simulink model "Classic_Sawmill"  (R2024b)
settings: Solver=FixedStepAuto  StartTime=0.0  StopTime=Tsim  FixedStep=dT  RelTol=1e-3
values from neighbouring files (symbols this model uses):
  b = t + 2*s    (= 3.6)    [ParametriSegheria.m]    (also in ParametriSegheriaDinamica.m; main_param_CLASSIC.m; main_param_SCADA.m)
  change_cost = 60    [ParametriSegheriaDinamica.m]    (also in main_param_CLASSIC.m = 50; main_param_SCADA.m = 50)
  dT = 0.025    [ParametriSegheriaDinamica.m]    (also in main_param_CLASSIC.m; main_param_SCADA.m)
  h_index = [70, 80, 90, 100]    [ParametriSegheria.m]    (also in ParametriSegheriaDinamica.m = [80, 90, 100]; main_param_CLASSIC.m = [80, 90, 100, 110]; main_param_SCADA.m = [80, 90, 100, 110])
  h_start_1 = 1    [main_param_CLASSIC.m]
  h_start_2 = 2    [main_param_CLASSIC.m]
  h_start_3 = 3    [main_param_CLASSIC.m]
  h_start_4 = 1    [main_param_CLASSIC.m]
  h_start_5 = 2    [main_param_CLASSIC.m]
  h_start_6 = 3    [main_param_CLASSIC.m]
  J1 = 8*1e6    (= 8000000)    [ParametriSegheriaDinamica.m]    (also in main_param_CLASSIC.m; main_param_SCADA.m)
  J2 = 0.9*1e6    (= 900000)    [ParametriSegheriaDinamica.m]    (also in main_param_CLASSIC.m; main_param_SCADA.m)
  kc = [0 35 40 50 55 90]    [ParametriSegheria.m]    (also in ParametriSegheriaDinamica.m = [0, 25, 30, 35, 50, 70]; main_param_CLASSIC.m = [0, 25, 30, 35, 50, 70]; main_param_SCADA.m = [0, 25, 30, 35, 50, 70])
  Kt = 2    [ParametriSegheria.m]    (also in ParametriSegheriaDinamica.m = 10000; main_param_CLASSIC.m = 10000; main_param_SCADA.m = 10000)
  Kt2 = 5    [ParametriSegheria.m]    (also in ParametriSegheriaDinamica.m = 4500; main_param_CLASSIC.m = 4500; main_param_SCADA.m = 4500)
  l_index = [20, 30, 40, 50]    [ParametriSegheria.m]    (also in ParametriSegheriaDinamica.m = [30, 40, 50]; main_param_CLASSIC.m = [30, 40, 50, 60]; main_param_SCADA.m = [30, 40, 50, 60])
  l_start_1 = 1    [main_param_CLASSIC.m]
  l_start_2 = 1    [main_param_CLASSIC.m]
  l_start_3 = 1    [main_param_CLASSIC.m]
  l_start_4 = 1    [main_param_CLASSIC.m]
  l_start_5 = 1    [main_param_CLASSIC.m]
  l_start_6 = 1    [main_param_CLASSIC.m]
  Lt = 4    [ParametriSegheria.m]    (also in ParametriSegheriaDinamica.m; main_param_CLASSIC.m; main_param_SCADA.m)
  Mag_D1 = [0 randi([220 500], 1, 40)]    [ParametriSegheria.m]    (also in ParametriSegheriaDinamica.m = [0 randi([200 500], 1, N_log)]; main_param_CLASSIC.m = [0 randi([200 500], 1, N_log)]; main_param_SCADA.m = [0 randi([200 500], 1, N_log)])
  Mag_D2 = [0 randi([220 500], 1, 40)]    [ParametriSegheria.m]    (also in ParametriSegheriaDinamica.m = [0 randi([200 500], 1, N_log)]; main_param_CLASSIC.m = [0 randi([200 500], 1, N_log)]; main_param_SCADA.m = [0 randi([200 500], 1, N_log)])
  Mag_D3 = [0 randi([220 500], 1, 40)]    [ParametriSegheria.m]    (also in ParametriSegheriaDinamica.m = [0 randi([200 500], 1, N_log)]; main_param_CLASSIC.m = [0 randi([200 500], 1, N_log)]; main_param_SCADA.m = [0 randi([200 500], 1, N_log)])
  Mag_legno1 = [0 randi([1 5], 1, 40)]    [ParametriSegheria.m]    (also in ParametriSegheriaDinamica.m = [0 randi([1 5], 1, N_log)]; main_param_CLASSIC.m = [0 randi([1 5], 1, N_log)]; main_param_SCADA.m = [0 randi([1 5], 1, N_log)])
  Mag_legno2 = [0 randi([1 5], 1, 40)]    [ParametriSegheria.m]    (also in ParametriSegheriaDinamica.m = [0 randi([1 5], 1, N_log)]; main_param_CLASSIC.m = [0 randi([1 5], 1, N_log)]; main_param_SCADA.m = [0 randi([1 5], 1, N_log)])
  Mag_legno3 = [0 randi([1 5], 1, 40)]    [ParametriSegheria.m]    (also in ParametriSegheriaDinamica.m = [0 randi([1 5], 1, N_log)]; main_param_CLASSIC.m = [0 randi([1 5], 1, N_log)]; main_param_SCADA.m = [0 randi([1 5], 1, N_log)])
  n_linee = 3    [ParametriSegheriaDinamica.m]    (also in main_param_CLASSIC.m; main_param_SCADA.m)
  omega_ref1 = 50    [ParametriSegheriaDinamica.m]    (also in main_param_CLASSIC.m; main_param_SCADA.m)
  omega_ref2 = 3000*(2*pi/60)    (= 314.159265359)    [ParametriSegheriaDinamica.m]    (also in main_param_CLASSIC.m; main_param_SCADA.m)
  Rc = 200    [ParametriSegheria.m]    (also in ParametriSegheriaDinamica.m; main_param_CLASSIC.m; main_param_SCADA.m)
  rho = [0, 450, 520, 590, 710, 780]*1e-9    [ParametriSegheriaDinamica.m]    (also in main_param_CLASSIC.m; main_param_SCADA.m)
  Rs = 800    [ParametriSegheria.m]    (also in ParametriSegheriaDinamica.m; main_param_CLASSIC.m; main_param_SCADA.m)
  sigma_D = 10    [ParametriSegheriaDinamica.m]    (also in main_param_CLASSIC.m = 5; main_param_SCADA.m = 5)
  sigma_larg = 10    [ParametriSegheriaDinamica.m]    (also in main_param_CLASSIC.m = 5; main_param_SCADA.m = 5)
  SR = Rs/Rm    (= 5.33333333333)    [ParametriSegheria.m]    (also in ParametriSegheriaDinamica.m; main_param_CLASSIC.m; main_param_SCADA.m)
  SR2 = Rc/Rm2    (= 4)    [ParametriSegheria.m]    (also in ParametriSegheriaDinamica.m; main_param_CLASSIC.m; main_param_SCADA.m)
  target_matrice = randi([20, 120], length(h_index), length(l_index))    [ParametriSegheria.m]    (also in ParametriSegheriaDinamica.m = randi([20, 100], length(h_index), length(l_index)); main_param_CLASSIC.m = randi([20, 100], length(h_index), length(l_index)); main_param_SCADA.m = randi([20, 100], length(h_index), length(l_index)))
  thr_lavoro = 600000    [ParametriSegheriaDinamica.m]    (also in main_param_CLASSIC.m; main_param_SCADA.m)
  V_mean1 = 0.75    [ParametriSegheriaDinamica.m]    (also in main_param_CLASSIC.m; main_param_SCADA.m)
  V_mean23 = 1    [ParametriSegheriaDinamica.m]    (also in main_param_CLASSIC.m; main_param_SCADA.m)
libraries: simulink x24, slpidlib x18
(part 4 of 5)

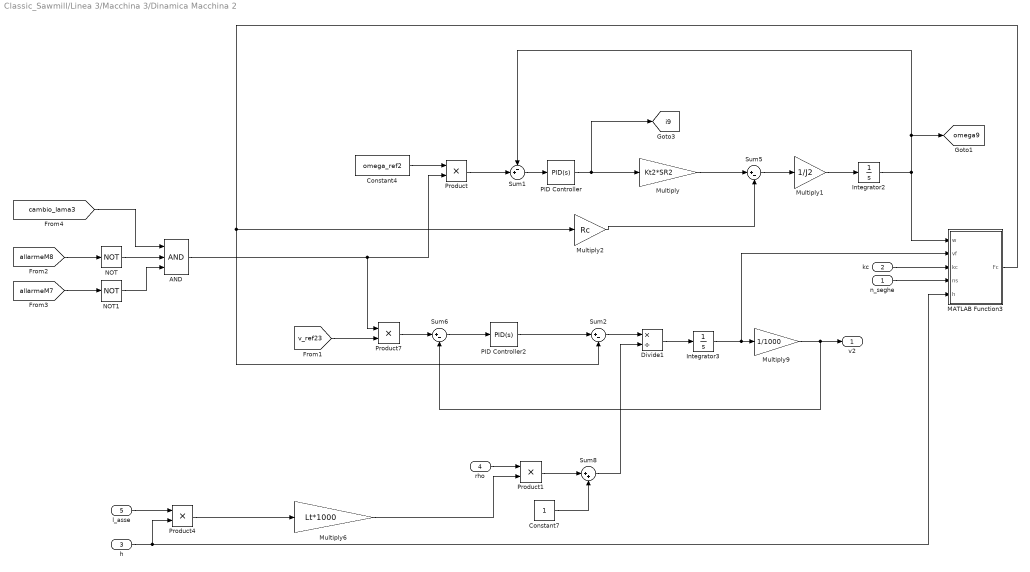
== system Classic_Sawmill/Linea 3/Macchina 3/Dinamica Macchina 2 ==
  n_seghe : Inport
  kc : Inport  Port=2
  h : Inport  Port=3
  rho : Inport  Port=4
  l_asse : Inport  Port=5
  AND : Logic  Inputs=3  IconShape=distinctive  AllPortsSameDT=off  OutDataTypeStr=boolean
  Constant4 : Constant  Value=omega_ref2
  Constant7 : Constant
  Divide1 : Product  Inputs=*/
  Integrator2 : Integrator  InitialCondition=omega_ref2
  Integrator3 : Integrator  InitialCondition=V_mean23*1000
  MATLAB Function3 : MATLAB Function  TreatAsAtomicUnit=on
  Multiply : Gain  Gain=Kt2*SR2
  Multiply1 : Gain  Gain=1/J2
  Multiply2 : Gain  Gain=Rc
  Multiply6 : Gain  Gain=Lt*1000
  Multiply9 : Gain  Gain=1/1000
  NOT : Logic  Operator=NOT  IconShape=distinctive  AllPortsSameDT=off  OutDataTypeStr=boolean
  NOT1 : Logic  Operator=NOT  IconShape=distinctive  AllPortsSameDT=off  OutDataTypeStr=boolean
  PID Controller : slpidlib/PID Controller  Controller=PID  Form=Parallel  TimeDomain=Continuous-time  UseExternalTs=off  SampleTime=-1  IntegratorMethod=Forward Euler  FilterMethod=Forward Euler  ControllerParametersSource=internal  P=345.484777327525  I=442.07289174245  UseKiTs=off  D=9.05690517196235  UseExternalDerivativeSource=off  N=26.4189049403583  UseFilter=on  TunerSelectOption=Transfer Function Based (PID Tuner App)  InitialConditionSource=internal  InitialConditionForIntegrator=0  InitialConditionForFilter=0  DifferentiatorICPrevScaledInput=0  ExternalReset=none  TrackingMode=off  Kt=1  LimitOutput=on  SatLimitsSource=internal  UpperSaturationLimit=300  LowerSaturationLimit=-300  LinearizeAsGain=on  AntiWindupMode=clamping  Kb=1  LimitIntegrator=off  UpperIntegratorSaturationLimit=200  LowerIntegratorSaturationLimit=-inf  POutMin=[]  POutMax=[]  IOutMin=[]  IOutMax=[]  DOutMin=[]  DOutMax=[]  NOutMin=[]  NOutMax=[]  SumOutMin=[]  SumOutMax=[]  SaturationOutMin=[]  SaturationOutMax=[]  PParamMin=[]  PParamMax=[]  IParamMin=[]  IParamMax=[]  DParamMin=[]  DParamMax=[]  NParamMin=[]  NParamMax=[]  KbParamMin=[]  KbParamMax=[]  KtParamMin=[]  KtParamMax=[]  KbOutMin=[]  KbOutMax=[]  KtOutMin=[]  KtOutMax=[]  IntegratorOutMin=[]  IntegratorOutMax=[]  FilterOutMin=[]  FilterOutMax=[]  SumI1OutMin=[]  SumI1OutMax=[]  SumI2OutMin=[]  SumI2OutMax=[]  SumI3OutMin=[]  SumI3OutMax=[]  SumI4OutMin=[]  SumI4OutMax=[]  SumDOutMin=[]  SumDOutMax=[]  DifferentiatorOutMin=[]  DifferentiatorOutMax=[]  FilterDiffOutCoefMin=[]  FilterDiffOutCoefMax=[]  ReciprocalOutMin=[]  ReciprocalOutMax=[]  SumDenOutMin=[]  SumDenOutMax=[]  SumNumOutMin=[]  SumNumOutMax=[]  DivideOutMin=[]  DivideOutMax=[]  UdiffTsProdOutMin=[]  UdiffTsProdOutMax=[]  NTsProdOutMin=[]  NTsProdOutMax=[]  UintegralTsProdOutMin=[]  UintegralTsProdOutMax=[]  UngainTsProdOutMin=[]  UngainTsProdOutMax=[]  ClampingZeroOutDataTypeStr=Inherit: Inherit via back propagation  ClampingZeroOutMin=[]  ClampingZeroOutMax=[]  FilterDenConstantOutDataTypeStr=Inherit: Inherit via back propagation  FilterDenConstantOutMin=[]  FilterDenConstantOutMax=[]  PCopyOutDataTypeStr=Inherit: Inherit via back propagation  PCopyOutMin=[]  PCopyOutMax=[]  NCopyOutDataTypeStr=Inherit: Inherit via back propagation  NCopyOutMin=[]  NCopyOutMax=[]  IntegratorContinuousStateAttributes=''  IntegratorStateMustResolveToSignalObject=off  IntegratorRTWStateStorageClass=Auto  FilterContinuousStateAttributes=''  FilterStateMustResolveToSignalObject=off  FilterRTWStateStorageClass=Auto  ParallelPVariant=InternalParameters  IdealPVariant=Disabled  IVariant=InternalParameters  DVariant=InternalParameters  IntegratorVariant=Continuous  SatVariant=Enabled  AWVariant=ContClampingParallel  PCopyVariant=Disabled  TRVariant=Disabled  FdbkBlocksVariant=Forward  IdealPFdbkVariant=Disabled  SatFdbkVariant=Disabled  DerivativeFilterVariant=ContFilter  NVariant=InternalParameters  NCopyVariant=Disabled  FilterICVariant=InternalICsFilter  IntegratorICVariant=InternalICs  ExternalResetVariant=Disabled  TRSumVariant=Passthrough  SumFdbkVariant=Disabled  SumVariant=Sum_PID  TsampFilterVariant=InternalTs  TsampNgainVariant=Passthrough  TsampIntegralVariant=Disabled_SignalSpec  ExternalSaturationOutDataTypeStr=Inherit: Same as second input  DerivativeSourceVariant=ErrorSignal  PreIntVariant=InternalPreInt
  PID Controller2 : slpidlib/PID Controller  Controller=PID  Form=Parallel  TimeDomain=Continuous-time  UseExternalTs=off  SampleTime=-1  IntegratorMethod=Forward Euler  FilterMethod=Forward Euler  ControllerParametersSource=internal  P=20866.9469532593  I=80635.0538109051  UseKiTs=off  D=181.138103439247  UseExternalDerivativeSource=off  N=79.7838174257724  UseFilter=on  TunerSelectOption=Transfer Function Based (PID Tuner App)  InitialConditionSource=internal  InitialConditionForIntegrator=0  InitialConditionForFilter=0  DifferentiatorICPrevScaledInput=0  ExternalReset=none  TrackingMode=off  Kt=1  LimitOutput=on  SatLimitsSource=internal  UpperSaturationLimit=5000  LowerSaturationLimit=-5000  LinearizeAsGain=off  AntiWindupMode=clamping  Kb=1  LimitIntegrator=off  UpperIntegratorSaturationLimit=200  LowerIntegratorSaturationLimit=-inf  POutMin=[]  POutMax=[]  IOutMin=[]  IOutMax=[]  DOutMin=[]  DOutMax=[]  NOutMin=[]  NOutMax=[]  SumOutMin=[]  SumOutMax=[]  SaturationOutMin=[]  SaturationOutMax=[]  PParamMin=[]  PParamMax=[]  IParamMin=[]  IParamMax=[]  DParamMin=[]  DParamMax=[]  NParamMin=[]  NParamMax=[]  KbParamMin=[]  KbParamMax=[]  KtParamMin=[]  KtParamMax=[]  KbOutMin=[]  KbOutMax=[]  KtOutMin=[]  KtOutMax=[]  IntegratorOutMin=[]  IntegratorOutMax=[]  FilterOutMin=[]  FilterOutMax=[]  SumI1OutMin=[]  SumI1OutMax=[]  SumI2OutMin=[]  SumI2OutMax=[]  SumI3OutMin=[]  SumI3OutMax=[]  SumI4OutMin=[]  SumI4OutMax=[]  SumDOutMin=[]  SumDOutMax=[]  DifferentiatorOutMin=[]  DifferentiatorOutMax=[]  FilterDiffOutCoefMin=[]  FilterDiffOutCoefMax=[]  ReciprocalOutMin=[]  ReciprocalOutMax=[]  SumDenOutMin=[]  SumDenOutMax=[]  SumNumOutMin=[]  SumNumOutMax=[]  DivideOutMin=[]  DivideOutMax=[]  UdiffTsProdOutMin=[]  UdiffTsProdOutMax=[]  NTsProdOutMin=[]  NTsProdOutMax=[]  UintegralTsProdOutMin=[]  UintegralTsProdOutMax=[]  UngainTsProdOutMin=[]  UngainTsProdOutMax=[]  ClampingZeroOutDataTypeStr=Inherit: Inherit via back propagation  ClampingZeroOutMin=[]  ClampingZeroOutMax=[]  FilterDenConstantOutDataTypeStr=Inherit: Inherit via back propagation  FilterDenConstantOutMin=[]  FilterDenConstantOutMax=[]  PCopyOutDataTypeStr=Inherit: Inherit via back propagation  PCopyOutMin=[]  PCopyOutMax=[]  NCopyOutDataTypeStr=Inherit: Inherit via back propagation  NCopyOutMin=[]  NCopyOutMax=[]  IntegratorContinuousStateAttributes=''  IntegratorStateMustResolveToSignalObject=off  IntegratorRTWStateStorageClass=Auto  FilterContinuousStateAttributes=''  FilterStateMustResolveToSignalObject=off  FilterRTWStateStorageClass=Auto  ParallelPVariant=InternalParameters  IdealPVariant=Disabled  IVariant=InternalParameters  DVariant=InternalParameters  IntegratorVariant=Continuous  SatVariant=Enabled  AWVariant=ContClampingParallel  PCopyVariant=Disabled  TRVariant=Disabled  FdbkBlocksVariant=Forward  IdealPFdbkVariant=Disabled  SatFdbkVariant=Disabled  DerivativeFilterVariant=ContFilter  NVariant=InternalParameters  NCopyVariant=Disabled  FilterICVariant=InternalICsFilter  IntegratorICVariant=InternalICs  ExternalResetVariant=Disabled  TRSumVariant=Passthrough  SumFdbkVariant=Disabled  SumVariant=Sum_PID  TsampFilterVariant=InternalTs  TsampNgainVariant=Passthrough  TsampIntegralVariant=Disabled_SignalSpec  ExternalSaturationOutDataTypeStr=Inherit: Same as second input  DerivativeSourceVariant=ErrorSignal  PreIntVariant=InternalPreInt
  Product{,1,4,7} (4 alike) : Product
  Sum1 : Sum  Inputs=-+|
  Sum2 : Sum  Inputs=|+-
  Sum5 : Sum  Inputs=|+-
  Sum6 : Sum  Inputs=|+-
  Sum8 : Sum  Inputs=|++
  v2 : Outport
  tag scope: i9=global, omega9=global
  wires:
  Product4/1 -> Multiply6/1
  h/1 -> MATLAB Function3/5(h), Product4/2
  l_asse/1 -> Product4/1
  Constant4/1 -> Product/1
  [v_ref23] -> Product7/2
  Product/1 -> Sum1/2
  Sum1/1 -> PID Controller/1
  rho/1 -> Product1/1
  AND/1 -> Product/2, Product7/1
  Sum5/1 -> Multiply1/1
  Multiply1/1 -> Integrator2/1
  PID Controller/1 -> [i9], Multiply/1
  MATLAB Function3/1(Fc) -> Sum2/2, Multiply2/1
  Sum6/1 -> PID Controller2/1
  Divide1/1 -> Integrator3/1
  Integrator3/1 -> MATLAB Function3/2(vf), Multiply9/1
  PID Controller2/1 -> Sum2/1
  Integrator2/1 -> MATLAB Function3/1(w), [omega9], Sum1/1
  Sum2/1 -> Divide1/1
  Product7/1 -> Sum6/1
  kc/1 -> MATLAB Function3/3(kc)
  Multiply6/1 -> Product1/2
  n_seghe/1 -> MATLAB Function3/4(ns)
  Product1/1 -> Sum8/1
  Sum8/1 -> Divide1/2
  Constant7/1 -> Sum8/2
  Multiply9/1 -> v2/1, Sum6/2
  Multiply/1 -> Sum5/1
  Multiply2/1 -> Sum5/2
  NOT1/1 -> AND/3
  [allarmeM8] -> NOT/1
  [allarmeM7] -> NOT1/1
  NOT/1 -> AND/2
  [cambio_lama3] -> AND/1

== matlab function Classic_Sawmill/Linea 1/MATLAB Function1 ==
  data: u input; y output
function y = fcn(u)

    persistent n_prec

    if isempty(n_prec)
        n_prec = 0;
    end

    y = u - n_prec;

    n_prec = u;

== matlab function Classic_Sawmill/Controllo Magazzino/MATLAB Function4 ==
  data: u input; idx output; h_index parameter
function idx = find_index(u, h_index)
%#codegen

v = h_index;

idx = -1; % valore default se non trovato

for i = 1:length(v)
    if u == v(i)
        idx = i;
        return;
    end
end

== matlab function Classic_Sawmill/Controllo Magazzino/MATLAB Function5 ==
  data: u input; idx output; l_index parameter
function idx = find_index(u, l_index)
%#codegen

v = l_index;

idx = -1; % valore default se non trovato

for i = 1:length(v)
    if u == v(i)
        idx = i;
        return;
    end
end

== matlab function Classic_Sawmill/Linea 2/MATLAB Function ==
  data: u input; y output
function y = fcn(u)

    persistent n_prec

    if isempty(n_prec)
        n_prec = 0;
    end

    y = u - n_prec;


    n_prec = u;

== matlab function Classic_Sawmill/Linea 2/MATLAB Function1 ==
  data: u input; y output
function y = fcn(u)

    persistent n_prec

    if isempty(n_prec)
        n_prec = 0;
    end

    y = u - n_prec;

    n_prec = u;

== matlab function Classic_Sawmill/Linea 2/MATLAB Function2 ==
  settings: updateMethod=DISCRETE
  data: lama_usurata input; y output; tronco_finito input
function y = fcn(lama_usurata, tronco_finito)
    
    persistent cambia_lama
    if isempty(cambia_lama)
        cambia_lama = 0;
    end

    if lama_usurata == 1
        cambia_lama = 1;
    end

    if tronco_finito == 1 && cambia_lama == 1
        y = cambia_lama;
        cambia_lama = 0;
    else
        y = 0;
    end

== matlab function Classic_Sawmill/Linea 2/MATLAB Function3 ==
  settings: updateMethod=DISCRETE
  data: u input; y output; t input; tempo_cambio parameter
function y = f(u, t, tempo_cambio)
persistent t_start active

if isempty(active)
    active = false;
    t_start = 0;
end

if u == 1 && ~active
    t_start = t;
    active = true;
end

if active
    if (t - t_start) <= tempo_cambio
        y = 0;
    else
        y = 1;
        active = false;
    end
else
    y = 1;
end

== matlab function Classic_Sawmill/Linea 2/Macchina 1/Dinamica Macchina 1/MATLAB Function3 ==
  data: w input; Fc output; vf input; kc input; Dt input; Rs parameter; b parameter
function Fc = Fcfun(w, vf, kc, Dt, Rs, b)

if w < 0.01
    Fc = 0;
else
    Fc = kc*b*vf*Dt/(w*Rs);
end

== matlab function Classic_Sawmill/Linea 2/Macchina 1/Logica Macchina 1/MATLAB Function ==
  data: u input; y output; Mag_legno2 parameter
function y = fcn(u, Mag_legno2)
    persistent counter
    if isempty(counter)
        counter = 1;
    end

    if u == 1
        counter = counter + 1;
    end

    y = counter;
    
    if y > length(Mag_legno2)-1
        y = 0;
    end

end

== matlab function Classic_Sawmill/Linea 3/MATLAB Function ==
  data: u input; y output
function y = fcn(u)

    persistent n_prec

    if isempty(n_prec)
        n_prec = 0;
    end

    y = u - n_prec;


    n_prec = u;

== matlab function Classic_Sawmill/Linea 3/MATLAB Function1 ==
  data: u input; y output
function y = fcn(u)

    persistent n_prec

    if isempty(n_prec)
        n_prec = 0;
    end

    y = u - n_prec;

    n_prec = u;

== matlab function Classic_Sawmill/Linea 3/MATLAB Function2 ==
  settings: updateMethod=DISCRETE
  data: lama_usurata input; y output; tronco_finito input
function y = fcn(lama_usurata, tronco_finito)
    
    persistent cambia_lama
    if isempty(cambia_lama)
        cambia_lama = 0;
    end

    if lama_usurata == 1
        cambia_lama = 1;
    end

    if tronco_finito == 1 && cambia_lama == 1
        y = cambia_lama;
        cambia_lama = 0;
    else
        y = 0;
    end

== matlab function Classic_Sawmill/Linea 3/MATLAB Function3 ==
  settings: updateMethod=DISCRETE
  data: u input; y output; t input; tempo_cambio parameter
function y = f(u, t,tempo_cambio)
persistent t_start active

if isempty(active)
    active = false;
    t_start = 0;
end

if u == 1 && ~active
    t_start = t;
    active = true;
end

if active
    if (t - t_start) <= tempo_cambio
        y = 0;
    else
        y = 1;
        active = false;
    end
else
    y = 1;
end

== matlab function Classic_Sawmill/Linea 3/Macchina 1/Dinamica Macchina 1/MATLAB Function3 ==
  data: w input; Fc output; vf input; kc input; Dt input; Rs parameter; b parameter
function Fc = Fcfun(w, vf, kc, Dt, Rs, b)

if w < 0.01
    Fc = 0;
else
    Fc = kc*b*vf*Dt/(w*Rs);
end

== matlab function Classic_Sawmill/Linea 3/Macchina 1/Logica Macchina 1/MATLAB Function ==
  data: u input; y output; Mag_legno3 parameter
function y = fcn(u, Mag_legno3)
    persistent counter
    if isempty(counter)
        counter = 1;
    end

    if u == 1
        counter = counter + 1;
    end

    y = counter;
    
    if y > length(Mag_legno3)-1
        y = 0;
    end

end

== matlab function Classic_Sawmill/Controllo Magazzino/MATLAB Function6 ==
  data: u input; idx output; h_index parameter
function idx = find_index(u, h_index)
%#codegen

v = h_index;

idx = -1; % valore default se non trovato

for i = 1:length(v)
    if u == v(i)
        idx = i;
        return;
    end
end

== matlab function Classic_Sawmill/Controllo Magazzino/MATLAB Function7 ==
  data: u input; idx output; h_index parameter
function idx = find_index(u, h_index)
%#codegen

v = h_index;

idx = -1; % valore default se non trovato

for i = 1:length(v)
    if u == v(i)
        idx = i;
        return;
    end
end

== matlab function Classic_Sawmill/Controllo Magazzino/MATLAB Function8 ==
  data: u input; idx output; h_index parameter
function idx = find_index(u, h_index)
%#codegen

v = h_index;

idx = -1; % valore default se non trovato

for i = 1:length(v)
    if u == v(i)
        idx = i;
        return;
    end
end

== matlab function Classic_Sawmill/Controllo Magazzino/MATLAB Function9 ==
  data: u input; idx output; h_index parameter
function idx = find_index(u, h_index)
%#codegen

v = h_index;

idx = -1; % valore default se non trovato

for i = 1:length(v)
    if u == v(i)
        idx = i;
        return;
    end
end

== matlab function Classic_Sawmill/Controllo Magazzino/MATLAB Function10 ==
  data: u input; idx output; l_index parameter
function idx = find_index(u, l_index)
%#codegen

v = l_index;

idx = -1; % valore default se non trovato

for i = 1:length(v)
    if u == v(i)
        idx = i;
        return;
    end
end

== matlab function Classic_Sawmill/Controllo Magazzino/MATLAB Function11 ==
  data: u input; idx output; l_index parameter
function idx = find_index(u, l_index)
%#codegen

v = l_index;

idx = -1; % valore default se non trovato

for i = 1:length(v)
    if u == v(i)
        idx = i;
        return;
    end
end

== matlab function Classic_Sawmill/Controllo Magazzino/MATLAB Function12 ==
  data: u input; idx output; l_index parameter
function idx = find_index(u, l_index)
%#codegen

v = l_index;

idx = -1; % valore default se non trovato

for i = 1:length(v)
    if u == v(i)
        idx = i;
        return;
    end
end

== matlab function Classic_Sawmill/Controllo Magazzino/MATLAB Function13 ==
  data: u input; idx output; l_index parameter
function idx = find_index(u, l_index)
%#codegen

v = l_index;

idx = -1; % valore default se non trovato

for i = 1:length(v)
    if u == v(i)
        idx = i;
        return;
    end
end

== matlab function Classic_Sawmill/Controllo Magazzino/INTELLIGENTE ==
  data: h_next output; Magazzino output; stop output; l_next output; h_idx input; target_matrice parameter; n_assi input; l_idx input; change_cost parameter; flag output
function [h_next, Magazzino, stop, l_next, flag] = fcn(h_idx, target_matrice, n_assi, l_idx, change_cost)

[n_rows, n_cols] = size(target_matrice);

h_next = zeros(1,length(h_idx));
l_next = zeros(1,length(l_idx));

persistent MagazzinoReale



if isempty(MagazzinoReale)
    MagazzinoReale = zeros(n_rows, n_cols);
end

for i = 1:length(n_assi)
    % Output iniziali
    h_next(i) = h_idx(i);
    l_next(i) = l_idx(i);
    

    MagazzinoReale(h_idx(i), l_idx(i)) = MagazzinoReale(h_idx(i), l_idx(i)) + n_assi(i);
end
    

% AVVISO QUANDO STO PER FINIRE QUELLA SEZIONE
thr = 10;
diff = zeros(1, length(n_assi));
flag = zeros(1, length(n_assi));

for i = 1:length(n_assi)
    diff(i) = target_matrice(h_idx(i), l_idx(i)) - MagazzinoReale(h_idx(i), l_idx(i));
    if diff(i) <= thr
        flag(i) = 1;
    else 
        flag(i) = 0;
    end
end



for i = 1:length(n_assi)
    if MagazzinoReale(h_idx(i), l_idx(i)) >= target_matrice(h_idx(i), l_idx(i)) + 1


        deficit = target_matrice - MagazzinoReale;

        best_cost = inf;
        best_h = h_idx(i);
        best_l = l_idx(i);

        
        for h = 1:n_rows
            for l = 1:n_cols

                if deficit(h,l) > 0

                    % Penalità cambio lama
                    if mod(i, 2) == 0
                        cambio = (h ~= h_idx(i));
                    else
                        cambio = (l ~= l_idx(i));
                    end

                    % Funzione costo
                    cost = -deficit(h,l) + change_cost*cambio;

                    if cost < best_cost
                        best_cost = cost;
                        best_h = h;
                        best_l = l;
                    end
                end

            end
        end

        if best_cost < inf
            h_next(i) = best_h;
            l_next(i) = best_l;
        end

    end
end

if MagazzinoReale >= target_matrice
    stop = 1;
else
    stop = 0;
end

Magazzino = MagazzinoReale;

== matlab function Classic_Sawmill/Linea 3/Macchina 1/Logica Macchina 1/MATLAB Function2 ==
  settings: updateMethod=DISCRETE
  data: spessore input; u input; spessore2 input; diametro input; y output; larg_asse output; thickness output; finito output; prior output; likelihood output; posterior output; larg_stim output; sigma_post output; sigma_larg parameter; sigma_D parameter
function [y, larg_asse, thickness, finito, prior, likelihood, posterior, larg_stim, sigma_post]= fcn(spessore, u, spessore2, diametro, sigma_larg, sigma_D)
    
    persistent in_rnd
        
    if isempty(in_rnd)
        rng(42, "twister");
        in_rnd = true;
    end

    persistent counter

    persistent noise_D

    if isempty(noise_D)
        noise_D = sigma_D*randn();
    end
  
    thin_cut = 4;

    max_assi = floor((diametro-thin_cut*spessore2) / spessore);
    finito = 0;

    maxD = 1000;
    larg_vec = 0:maxD;

    prior = zeros(size(larg_vec));
    likelihood = zeros(size(larg_vec));
    posterior = zeros(size(larg_vec));

    if isempty(counter)
        counter = 0;
    end
    

    % Conto assi tagliate
    if u == 1
        counter = counter + 1;
    end

    % Quando finisco tronco segnalo e azzero counter
    if counter > max_assi + thin_cut
        finito = 1;
        counter = 0;
    end

    if finito ~= 0
        noise_D = sigma_D*randn();
    end
    
    if diametro > 0
        misure_D = diametro + noise_D;
    else
        misure_D = diametro;
    end

    % SISTEMARE INCERTEZZA: propagata da D in L
    if counter == 0
        larg_asse = 0;
        larg_asseD = 0;
        thickness = 0;
        sigma_largD = 0;
    elseif counter <= thin_cut/2
        distanza_bordo = counter * spessore2;
        larg_asse = sqrt((diametro)^2-(spessore2 + diametro - 2*distanza_bordo)^2);
        thickness = spessore2;
        % prior
        larg_asseD = sqrt(abs((misure_D)^2-(spessore2 + misure_D - 2*distanza_bordo)^2));
        sigma_largD = abs((2*distanza_bordo - spessore2)/sqrt((2*distanza_bordo - spessore2)*(-2*distanza_bordo + 2*diametro + spessore2)))*sigma_D;
    elseif counter > max_assi + thin_cut/2
        distanza_bordo = max_assi*spessore + (counter-max_assi)*spessore2;
        larg_asse = sqrt((diametro)^2-(spessore2 + diametro - 2*distanza_bordo)^2);
        thickness = spessore2;
        % prior
        larg_asseD = sqrt(abs((misure_D)^2-(spessore2 + misure_D - 2*distanza_bordo)^2));
        sigma_largD = abs((2*distanza_bordo - spessore2)/sqrt((2*distanza_bordo - spessore2)*(-2*distanza_bordo + 2*diametro + spessore2)))*sigma_D;
    else
        % Calcolo larghezza delle assi
        distanza_bordo = thin_cut/2 * spessore2 + (counter-thin_cut/2) * spessore;
        larg_asse = sqrt((diametro)^2-(spessore + diametro - 2*distanza_bordo)^2);
        thickness = spessore;
        % prior
        larg_asseD = sqrt(abs((misure_D)^2-(spessore + misure_D - 2*distanza_bordo)^2));
        sigma_largD = abs((2*distanza_bordo - spessore)/sqrt((2*distanza_bordo - spessore)*(-2*distanza_bordo + 2*diametro + spessore)))*sigma_D;
    end




    if larg_asse > 0
        misure_larg = larg_asse + sigma_larg * randn();
    else
        misure_larg = larg_asse;
    end

    if larg_asse > 0
        prior(:) = 1/sqrt(2*pi*sigma_largD^2)*exp(-0.5 * ((larg_vec - larg_asseD) / sigma_largD).^2);
        prior(:) = prior(:) / sum(prior(:));
    else
        prior(:) = 0;
    end

    if misure_larg > 0
        likelihood(:) = 1/sqrt(2*pi*sigma_larg^2)*exp(-0.5 * ((larg_vec - misure_larg) / sigma_larg).^2);
        likelihood(:) = likelihood(:) / sum(likelihood(:));
    else
        likelihood(:) = 0;
    end

    if misure_larg > 0 && larg_asse > 0
        posterior(:) = prior(:) .* likelihood(:);
        posterior(:) = posterior(:) / sum(posterior(:));
    else
        posterior(:) = 0;
    end



    [~, idx] = max(posterior(:)); 

    larg_stim = larg_vec(idx);
    % (sigma_likelihood^2*sigma_prior^2)/(sigma_likelihood^2 + sigma_prior^2)
    sigma_post = sqrt( (sigma_largD^2*sigma_larg^2) / (sigma_largD^2 + sigma_larg^2) );
    
    y = counter;

== matlab function Classic_Sawmill/Controllo Magazzino/CAMBIO LAME CONSUMATE ==
  data: n_assi input; y output; cambio_1 output; cambio_2 output; cambio_3 output; kc input; Lt parameter; b parameter; h input; lavoro_l output; thr_lavoro parameter
function [y, cambio_1, cambio_2, cambio_3, lavoro_l] = fcn(n_assi, kc, Lt, b,h, thr_lavoro)

    warning = zeros(1, length(n_assi));

    persistent usura_lama
    persistent lavoro_lama

    if isempty(usura_lama)
        usura_lama = zeros(1, length(n_assi));
    end

    if isempty(lavoro_lama)
        lavoro_lama = zeros(1, length(n_assi));
    end

    cambio_1 = 0;
    cambio_2 = 0;
    cambio_3 = 0;

    for i = 1:length(n_assi)
        
        % Ogni volta che arriva un certo numero di assi vuol dire che le
        % lame hanno appena fatto un taglio
        if n_assi(i) ~= 0
            usura_lama(i) = usura_lama(i) + 1;
            lavoro_lama(i) = lavoro_lama(i) + kc(i)*b*Lt*h(i);
        end
        
        if lavoro_lama(i) > thr_lavoro
            warning(i) = 1;
            lavoro_lama(i) = 0;
        end

        % i = 1 -> M2 Linea 1
        % i = 2 -> M3 Linea 1
        % i = 3 -> M2 Linea 2
        % i = 4 -> M3 Linea 2
        % i = 5 -> M2 Linea 3
        % i = 6 -> M2 Linea 3
        if (i == 1 || i == 2) && warning(i) == 1
            cambio_1 = 1;
        elseif (i == 3 || i == 4) && warning(i) == 1
            cambio_2 = 1;
        elseif (i == 5 || i == 6) && warning(i) == 1
            cambio_3 = 1;
        end

    end

    lavoro_l = lavoro_lama;

    y = warning;

== matlab function Classic_Sawmill/Linea 1/Macchina 2/Dinamica Macchina 2/MATLAB Function3 ==
  data: w input; Fc output; vf input; kc input; ns input; h input; Rs parameter; b parameter
function Fc = Fcfun(w, vf, kc, ns, h, Rs, b)

if w < 0.01
    Fc = 0;
else
    Fc = ns*kc*b*vf*h/(w*Rs);
end

== matlab function Classic_Sawmill/Linea 1/MATLAB Function3 ==
  settings: updateMethod=DISCRETE
  data: u input; y output; t input; tempo_cambio parameter
function y = f(u, t, tempo_cambio)
persistent t_start active

if isempty(active)
    active = false;
    t_start = 0;
end

if u == 1 && ~active
    t_start = t;
    active = true;
end

if active
    if (t - t_start) <= tempo_cambio
        y = 0;
    else
        y = 1;
        active = false;
    end
else
    y = 1;
end

== matlab function Classic_Sawmill/Linea 1/Macchina 1/Logica Macchina 1/MATLAB Function1 ==
  settings: updateMethod=DISCRETE
  data: spessore input; u input; spessore2 input; diametro input; y output; larg_asse output; thickness output; finito output; prior output; likelihood output; posterior output; larg_stim output; sigma_post output; sigma_larg parameter; sigma_D parameter; t input
function [y, larg_asse, thickness, finito, prior, likelihood, posterior, larg_stim, sigma_post]= fcn(spessore, u, spessore2, diametro, sigma_larg, sigma_D, t)
    
    persistent in_rnd
        
    if isempty(in_rnd)
        rng(42, "twister");
        in_rnd = true;
    end

    persistent counter

    persistent noise_D

    if isempty(noise_D)
        noise_D = sigma_D*randn();
    end
  
    thin_cut = 4;

    max_assi = floor((diametro-thin_cut*spessore2) / spessore);
    finito = 0;

    maxD = 1000;
    larg_vec = 0:maxD;

    prior = zeros(size(larg_vec));
    likelihood = zeros(size(larg_vec));
    posterior = zeros(size(larg_vec));

    if isempty(counter)
        counter = 0;
    end
    

    % Conto assi tagliate
    if u == 1
        counter = counter + 1;
    end

    % Quando finisco tronco segnalo e azzero counter
    if counter > max_assi + thin_cut
        finito = 1;
        counter = 0;
    end

    if finito ~= 0
        noise_D = sigma_D*randn();
    end
    
    if diametro > 0
        misure_D = diametro + noise_D;
    else
        misure_D = diametro;
    end

    % SISTEMARE INCERTEZZA: propagata da D in L
    if counter == 0
        larg_asse = 0;
        larg_asseD = 0;
        thickness = 0;
        sigma_largD = 0;
        distanza_bordo = 0;
    elseif counter <= thin_cut/2
        distanza_bordo = counter * spessore2;
        larg_asse = sqrt((diametro)^2-(spessore2 + diametro - 2*distanza_bordo)^2);
        thickness = spessore2;
        % prior
        larg_asseD = sqrt(abs((misure_D)^2-(spessore2 + misure_D - 2*distanza_bordo)^2));
        sigma_largD = abs((2*distanza_bordo - spessore2)/sqrt((2*distanza_bordo - spessore2)*(-2*distanza_bordo + 2*diametro + spessore2)))*sigma_D;
    elseif counter > max_assi + thin_cut/2
        distanza_bordo = max_assi*spessore + (counter-max_assi)*spessore2;
        larg_asse = sqrt((diametro)^2-(spessore2 + diametro - 2*distanza_bordo)^2);
        thickness = spessore2;
        % prior
        larg_asseD = sqrt(abs((misure_D)^2-(spessore2 + misure_D - 2*distanza_bordo)^2));
        sigma_largD = abs((2*distanza_bordo - spessore2)/sqrt((2*distanza_bordo - spessore2)*(-2*distanza_bordo + 2*diametro + spessore2)))*sigma_D;
    else
        % Calcolo larghezza delle assi
        distanza_bordo = thin_cut/2 * spessore2 + (counter-thin_cut/2) * spessore;
        larg_asse = sqrt((diametro)^2-(spessore + diametro - 2*distanza_bordo)^2);
        thickness = spessore;
        % prior
        larg_asseD = sqrt(abs((misure_D)^2-(spessore + misure_D - 2*distanza_bordo)^2));
        sigma_largD = abs((2*distanza_bordo - spessore)/sqrt((2*distanza_bordo - spessore)*(-2*distanza_bordo + 2*diametro + spessore)))*sigma_D;
    end


    sens_break = 0;

    if larg_asse > 0
        if t > 35 && t < 50 && sens_break
            misure_larg = larg_asse + sigma_larg * randn() + 100*rand;
        else
            misure_larg = larg_asse + sigma_larg * randn();
        end
    else
        misure_larg = larg_asse;
    end

    if larg_asse > 0
        prior(:) = 1/sqrt(2*pi*sigma_largD^2)*exp(-0.5 * ((larg_vec - larg_asseD) / sigma_largD).^2);
        prior(:) = prior(:) / sum(prior(:));
    else
        prior(:) = 0;
    end

    if misure_larg > 0
        likelihood(:) = 1/sqrt(2*pi*sigma_larg^2)*exp(-0.5 * ((larg_vec - misure_larg) / sigma_larg).^2);
        likelihood(:) = likelihood(:) / sum(likelihood(:));
    else
        likelihood(:) = 0;
    end

    if misure_larg > 0 && larg_asse > 0
        posterior(:) = prior(:) .* likelihood(:);
        posterior(:) = posterior(:) / sum(posterior(:));
    else
        posterior(:) = 0;
    end



    [~, idx] = max(posterior(:)); 

    larg_stim = larg_vec(idx);
    % (sigma_likelihood^2*sigma_prior^2)/(sigma_likelihood^2 + sigma_prior^2)
    sigma_post = sqrt( (sigma_largD^2*sigma_larg^2) / (sigma_largD^2 + sigma_larg^2) );
    
    y = counter;

== matlab function Classic_Sawmill/Linea 2/Macchina 2/Dinamica Macchina 2/MATLAB Function3 ==
  data: w input; Fc output; vf input; kc input; ns input; h input; Rs parameter; b parameter
function Fc = Fcfun(w, vf, kc, ns, h, Rs, b)

if w < 0.01
    Fc = 0;
else
    Fc = ns*kc*b*vf*h/(w*Rs);
end

== matlab function Classic_Sawmill/Linea 1/Macchina 2/MATLAB Function2 ==
  settings: updateMethod=DISCRETE
  data: u input; w_asse input; y output; l_asse input; taglio output; Lt parameter
function [y, taglio] = fcn(u, w_asse, l_asse,Lt)
    persistent counter 

    n_assi = floor(l_asse / w_asse);
    
    taglio = 0;

    if isempty(counter)
        counter = 0;
    end

    % Conto assi tagliate
    if u >= Lt
        counter = counter + n_assi;
    end

    % Segnale di taglio
    if  (u > 0 && u < Lt && l_asse > 0) 
        taglio = 1;
    end
    y = counter;
end

== matlab function Classic_Sawmill/Linea 3/Macchina 2/Dinamica Macchina 2/MATLAB Function3 ==
  data: w input; Fc output; vf input; kc input; ns input; h input; Rs parameter; b parameter
function Fc = Fcfun(w, vf, kc, ns, h, Rs, b)

if w < 0.01
    Fc = 0;
else
    Fc = ns*kc*b*vf*h/(w*Rs);
end

== matlab function Classic_Sawmill/Linea 1/Macchina 3/Dinamica Macchina 2/MATLAB Function3 ==
  data: w input; Fc output; vf input; kc input; ns input; h input; Rs parameter; b parameter
function Fc = Fcfun(w, vf, kc, ns, h, Rs, b)

if w < 0.01
    Fc = 0;
else
    Fc = ns*kc*b*vf*h/(w*Rs);
end

== matlab function Classic_Sawmill/Linea 1/Macchina 3/MATLAB Function2 ==
  settings: updateMethod=DISCRETE
  data: u input; w_asse input; y output; l_asse input; taglio output; Lt parameter
function [y, taglio] = fcn(u, w_asse, l_asse,Lt)
    persistent counter 

    n_assi = floor(l_asse / w_asse);
    
    taglio = 0;

    if isempty(counter)
        counter = 0;
    end

    % Conto assi tagliate
    if u >= Lt
        counter = counter + n_assi;
    end

    % Segnale di taglio
    if  (u > 0 && u < Lt && l_asse > 0) 
        taglio = 1;
    end
    y = counter;
end

== matlab function Classic_Sawmill/Linea 1/MATLAB Function2 ==
  settings: updateMethod=DISCRETE
  data: lama_usurata input; y output; tronco_finito input
function y = fcn(lama_usurata, tronco_finito)
    
    persistent cambia_lama
    if isempty(cambia_lama)
        cambia_lama = 0;
    end

    if lama_usurata == 1
        cambia_lama = 1;
    end

    if tronco_finito == 1 && cambia_lama == 1
        y = cambia_lama;
        cambia_lama = 0;
    else
        y = 0;
    end

== matlab function Classic_Sawmill/Linea 2/Macchina 2/MATLAB Function2 ==
  settings: updateMethod=DISCRETE
  data: u input; w_asse input; y output; l_asse input; taglio output; Lt parameter
function [y, taglio] = fcn(u, w_asse, l_asse,Lt)
    persistent counter 

    n_assi = floor(l_asse / w_asse);
    
    taglio = 0;

    if isempty(counter)
        counter = 0;
    end

    % Conto assi tagliate
    if u >= Lt
        counter = counter + n_assi;
    end

    % Segnale di taglio
    if  (u > 0 && u < Lt && l_asse > 0) 
        taglio = 1;
    end
    y = counter;
end

== matlab function Classic_Sawmill/Linea 2/Macchina 3/Dinamica Macchina 2/MATLAB Function3 ==
  data: w input; Fc output; vf input; kc input; ns input; h input; Rs parameter; b parameter
function Fc = Fcfun(w, vf, kc, ns, h, Rs, b)

if w < 0.01
    Fc = 0;
else
    Fc = ns*kc*b*vf*h/(w*Rs);
end

== matlab function Classic_Sawmill/Linea 1/Macchina 1/Logica Macchina 1/MATLAB Function ==
  data: u input; y output; Mag_legno1 parameter
function y = fcn(u, Mag_legno1)
    persistent counter
    if isempty(counter)
        counter = 1;
    end

    if u == 1
        counter = counter + 1;
    end

    y = counter;
    
    if y > length(Mag_legno1)-1
        y = 0;
    end

end

== matlab function Classic_Sawmill/Linea 2/Macchina 3/MATLAB Function2 ==
  settings: updateMethod=DISCRETE
  data: u input; w_asse input; y output; l_asse input; taglio output; Lt parameter
function [y, taglio] = fcn(u, w_asse, l_asse,Lt)
    persistent counter 

    n_assi = floor(l_asse / w_asse);
    
    taglio = 0;

    if isempty(counter)
        counter = 0;
    end

    % Conto assi tagliate
    if u >= Lt
        counter = counter + n_assi;
    end

    % Segnale di taglio
    if  (u > 0 && u < Lt && l_asse > 0) 
        taglio = 1;
    end
    y = counter;
end

== matlab function Classic_Sawmill/Linea 3/Macchina 2/MATLAB Function2 ==
  settings: updateMethod=DISCRETE
  data: u input; w_asse input; y output; l_asse input; taglio output; Lt parameter
function [y, taglio] = fcn(u, w_asse, l_asse,Lt)
    persistent counter 

    n_assi = floor(l_asse / w_asse);
    
    taglio = 0;

    if isempty(counter)
        counter = 0;
    end

    % Conto assi tagliate
    if u >= Lt
        counter = counter + n_assi;
    end

    % Segnale di taglio
    if  (u > 0 && u < Lt && l_asse > 0) 
        taglio = 1;
    end
    y = counter;
end

== matlab function Classic_Sawmill/Linea 3/Macchina 3/Dinamica Macchina 2/MATLAB Function3 ==
  data: w input; Fc output; vf input; kc input; ns input; h input; Rs parameter; b parameter
function Fc = Fcfun(w, vf, kc, ns, h, Rs, b)

if w < 0.01
    Fc = 0;
else
    Fc = ns*kc*b*vf*h/(w*Rs);
end

== matlab function Classic_Sawmill/Linea 3/Macchina 3/MATLAB Function2 ==
  settings: updateMethod=DISCRETE
  data: u input; w_asse input; y output; l_asse input; taglio output; Lt parameter
function [y, taglio] = fcn(u, w_asse, l_asse,Lt)
    persistent counter 

    n_assi = floor(l_asse / w_asse);
    
    taglio = 0;

    if isempty(counter)
        counter = 0;
    end

    % Conto assi tagliate
    if u >= Lt
        counter = counter + n_assi;
    end

    % Segnale di taglio
    if  (u > 0 && u < Lt && l_asse > 0) 
        taglio = 1;
    end
    y = counter;
end

== matlab function Classic_Sawmill/MATLAB Function ==
  data: v_ref1 output; v_ref23 output; n_attive input; n_linee parameter; V_mean1 parameter; V_mean23 parameter
function [v_ref1,v_ref23] = fcn(n_attive, n_linee, V_mean1, V_mean23)

if n_attive == 0
    v_ref1 = 0.01;
    v_ref23 = 0.01;
else
    % VELOCITA' NON DISTRIBUITE
    v_ref1 = V_mean1;
    v_ref23 = V_mean23;
end

== matlab function Classic_Sawmill/Controllo Magazzino/MATLAB Function ==
  data: true_n_assi input; n_assi_estimate output; lar_stim input; width_cut input; posterior output; likelihood output; prior output; sigma_larg input; k_cam parameter; sigma_cam output
function [n_assi_estimate, posterior, likelihood, prior, sigma_cam]= fcn(true_n_assi, lar_stim, width_cut, sigma_larg, k_cam)

    persistent in_rnd

    if isempty(in_rnd)
        rng(42, "twister");
        in_rnd = true;
    end
    
    n_assi_estimate = zeros(1, length(true_n_assi));
    misure_camera = zeros(1, length(true_n_assi));
    sigma_cam = zeros(1, length(true_n_assi));
   
    max_N = 30;         % Max boards number
    n_vec = 1:max_N;    % VEttore con tutti i numeri di assi possibili in output
    
    
    
    
    posterior = zeros(max_N, length(true_n_assi));
    likelihood = zeros(max_N, length(true_n_assi));
    prior = zeros(max_N, length(true_n_assi));

    

    for i = 1:length(true_n_assi)
        
        % SPORCO IL SEGNALE DI MISURA DELLA CAMERA 
        if true_n_assi(i) ~= 0
            if rand < 0.03
                if rand < 0.7
                    noise = -2;
                else 
                    noise = 2;
                end
            elseif rand < 0.1
                if rand < 0.7
                    noise = -1;
                else
                    noise = 1;
                end
            else
                noise = 0;
            end
        else
            noise = 0;
        end
        misure_camera(i) = true_n_assi(i) + noise;



        % Sigma dinamica che aumenta all'aumentare del numero di assi
        % misurate
        sigma_cam(i) = k_cam * misure_camera(i);

        if true_n_assi(i) ~= 0
        
            % Compute the prior (probability distribution for each board number
            % given that measure)
            % mu_larg = n_vec * width_cut(i); % + ((n_vec - 1) * t2);
            % prior(:, i) = exp(-0.5 * ((misure_larg(i) - mu_larg) / sigma_larg).^2);

            sigma_nl = sigma_larg(i)/width_cut(i);
            n_larg = floor(lar_stim(i)/width_cut(i));
            
            prior(:, i) = 1/sqrt(2*pi*sigma_nl^2)*exp(-0.5 * ((n_vec - n_larg) / sigma_nl).^2);
            prior(:, i) = prior(:, i) / sum(prior(:, i));

            % Initialize the likelihood from the camera sensor
            likelihood(:, i) = 1/sqrt(2*pi*sigma_cam(i)^2)*exp(-0.5 * ((n_vec - misure_camera(i)) / sigma_cam(i)).^2);
            likelihood(:, i) = likelihood(:, i) / sum(likelihood(:, i));
            
           

            % Compute the posterior - Bayesyan fusion
            % Riempio posteriori per ogni macchina così posso plottare la
            % distribuzione
            posterior(:, i) = prior(:, i) .* likelihood(:, i);
            posterior(:, i) = posterior(:, i) / sum(posterior(:, i));
            [~, idx] = max(posterior(:, i));


            n_assi_estimate(i) = n_vec(idx);
        else
            n_assi_estimate(i) = 0;
        end
    
    end

== matlab function Classic_Sawmill/Linea 2/Macchina 1/Logica Macchina 1/MATLAB Function2 ==
  settings: updateMethod=DISCRETE
  data: spessore input; u input; spessore2 input; diametro input; y output; larg_asse output; thickness output; finito output; prior output; likelihood output; posterior output; larg_stim output; sigma_post output; sigma_larg parameter; sigma_D parameter
function [y, larg_asse, thickness, finito, prior, likelihood, posterior, larg_stim, sigma_post]= fcn(spessore, u, spessore2, diametro, sigma_larg, sigma_D)
    
    persistent in_rnd
        
    if isempty(in_rnd)
        rng(42, "twister");
        in_rnd = true;
    end

    persistent counter

    persistent noise_D

    if isempty(noise_D)
        noise_D = sigma_D*randn();
    end
  
    thin_cut = 4;

    max_assi = floor((diametro-thin_cut*spessore2) / spessore);
    finito = 0;

    maxD = 1000;
    larg_vec = 0:maxD;

    prior = zeros(size(larg_vec));
    likelihood = zeros(size(larg_vec));
    posterior = zeros(size(larg_vec));

    if isempty(counter)
        counter = 0;
    end
    

    % Conto assi tagliate
    if u == 1
        counter = counter + 1;
    end

    % Quando finisco tronco segnalo e azzero counter
    if counter > max_assi + thin_cut
        finito = 1;
        counter = 0;
    end

    if finito ~= 0
        noise_D = sigma_D*randn();
    end
    
    if diametro > 0
        misure_D = diametro + noise_D;
    else
        misure_D = diametro;
    end

    % SISTEMARE INCERTEZZA: propagata da D in L
    if counter == 0
        larg_asse = 0;
        larg_asseD = 0;
        thickness = 0;
        sigma_largD = 0;
    elseif counter <= thin_cut/2
        distanza_bordo = counter * spessore2;
        larg_asse = sqrt((diametro)^2-(spessore2 + diametro - 2*distanza_bordo)^2);
        thickness = spessore2;
        % prior
        larg_asseD = sqrt(abs((misure_D)^2-(spessore2 + misure_D - 2*distanza_bordo)^2));
        sigma_largD = abs((2*distanza_bordo - spessore2)/sqrt((2*distanza_bordo - spessore2)*(-2*distanza_bordo + 2*diametro + spessore2)))*sigma_D;
    elseif counter > max_assi + thin_cut/2
        distanza_bordo = max_assi*spessore + (counter-max_assi)*spessore2;
        larg_asse = sqrt((diametro)^2-(spessore2 + diametro - 2*distanza_bordo)^2);
        thickness = spessore2;
        % prior
        larg_asseD = sqrt(abs((misure_D)^2-(spessore2 + misure_D - 2*distanza_bordo)^2));
        sigma_largD = abs((2*distanza_bordo - spessore2)/sqrt((2*distanza_bordo - spessore2)*(-2*distanza_bordo + 2*diametro + spessore2)))*sigma_D;
    else
        % Calcolo larghezza delle assi
        distanza_bordo = thin_cut/2 * spessore2 + (counter-thin_cut/2) * spessore;
        larg_asse = sqrt((diametro)^2-(spessore + diametro - 2*distanza_bordo)^2);
        thickness = spessore;
        % prior
        larg_asseD = sqrt(abs((misure_D)^2-(spessore + misure_D - 2*distanza_bordo)^2));
        sigma_largD = abs((2*distanza_bordo - spessore)/sqrt((2*distanza_bordo - spessore)*(-2*distanza_bordo + 2*diametro + spessore)))*sigma_D;
    end




    if larg_asse > 0
        misure_larg = larg_asse + sigma_larg * randn();
    else
        misure_larg = larg_asse;
    end

    if larg_asse > 0
        prior(:) = 1/sqrt(2*pi*sigma_largD^2)*exp(-0.5 * ((larg_vec - larg_asseD) / sigma_largD).^2);
        prior(:) = prior(:) / sum(prior(:));
    else
        prior(:) = 0;
    end

    if misure_larg > 0
        likelihood(:) = 1/sqrt(2*pi*sigma_larg^2)*exp(-0.5 * ((larg_vec - misure_larg) / sigma_larg).^2);
        likelihood(:) = likelihood(:) / sum(likelihood(:));
    else
        likelihood(:) = 0;
    end

    if misure_larg > 0 && larg_asse > 0
        posterior(:) = prior(:) .* likelihood(:);
        posterior(:) = posterior(:) / sum(posterior(:));
    else
        posterior(:) = 0;
    end



    [~, idx] = max(posterior(:)); 

    larg_stim = larg_vec(idx);
    % (sigma_likelihood^2*sigma_prior^2)/(sigma_likelihood^2 + sigma_prior^2)
    sigma_post = sqrt( (sigma_largD^2*sigma_larg^2) / (sigma_largD^2 + sigma_larg^2) );
    
    y = counter;

== matlab function Classic_Sawmill/Linea 1/Macchina 1/Dinamica Macchina 1/MATLAB Function3 ==
  data: w input; Fc output; vf input; kc input; Dt input; Rs parameter; b parameter
function Fc = Fcfun(w, vf, kc, Dt, Rs, b)

if w < 0.01
    Fc = 0;
else
    Fc = kc*b*vf*Dt/(w*Rs);
end

== matlab function Classic_Sawmill/Linea 1/MATLAB Function ==
  data: u input; y output
function y = fcn(u)

    persistent n_prec

    if isempty(n_prec)
        n_prec = 0;
    end

    y = u - n_prec;


    n_prec = u;

== matlab function Classic_Sawmill/Controllo Magazzino/MATLAB Function1 ==
  data: u input; idx output; h_index parameter
function idx = find_index(u, h_index)
%#codegen

v = h_index;

idx = -1; % valore default se non trovato

for i = 1:length(v)
    if u == v(i)
        idx = i;
        return;
    end
end

== matlab function Classic_Sawmill/Controllo Magazzino/MATLAB Function2 ==
  data: u input; idx output; l_index parameter
function idx = find_index(u, l_index)
%#codegen

v = l_index;

idx = -1; % valore default se non trovato

for i = 1:length(v)
    if u == v(i)
        idx = i;
        return;
    end
end
